simulink model "Scheme"  (R2015a)
settings: Solver=ode45  SolverMode=SingleTasking  StartTime=0.0  StopTime=10  RelTol=1e-3
libraries: simulink x1, dspsrcs4 x1
settings Model: CovSFcnEnable=off  Creator=Olia  LastModifiedBy=Windows 7
settings OptimizationCC: BlockReduction=off  BooleanDataType=off
settings DebuggingCC: SaveWithParameterizedLinksMsg=none  UnderspecifiedInitializationDetection=Classic  MergeDetectMultiDrivingBlocksExec=none  SignalResolutionControl=TryResolveAllWithWarning
settings HardwareCC: TargetUnknown=on

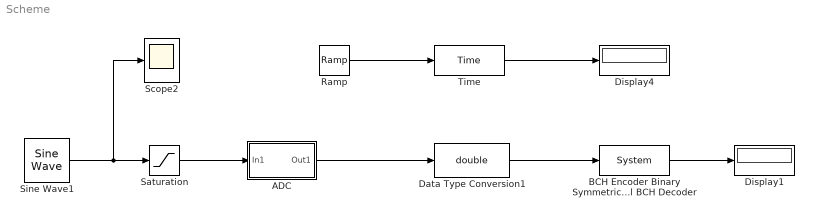
== system Scheme ==
  ADC : Subsystem
  BCH Encoder Binary Symmetric Channel BCH Decoder : MATLABFcn  MATLABFcn=System
  Data Type Conversion1 : DataTypeConversion  OutDataTypeStr=double
  Display1 : Display
  Display4 : Display
  Ramp : simulink/Sources/Ramp  slope=1  start=0  X0=0
  Saturation : Saturate  UpperLimit=2^24-1  LowerLimit=0
  Scope2 : Scope
      settings: TickLabels=on  YMin=0  YMax=10  SaveName=ScopeData2
  Sine Wave1 : dspsrcs4/Sine Wave  Amplitude=10  Frequency=2  Phase=0  SampleMode=Discrete  OutComplex=Real  CompMethod=Trigonometric fcn  TableSize=Speed  SampleTime=1/70  SamplesPerFrame=1  ResetState=Restart at time zero  dataType=double  wordLen=16  udDataType=sfix(16)  fracBitsMode=Best precision  numFracBits=15  OutDataTypeStr=double  LastOutDataTypeStr=double
  Time : MATLABFcn  MATLABFcn=Time
  wires:
  Sine Wave1/1 -> Saturation/1, Scope2/1
  Saturation/1 -> ADC/1(In1)
  ADC/1(Out1) -> Data Type Conversion1/1
  Time/1 -> Display4/1
  Ramp/1 -> Time/1
  Data Type Conversion1/1 -> BCH Encoder Binary Symmetric Channel BCH Decoder/1
  BCH Encoder Binary Symmetric Channel BCH Decoder/1 -> Display1/1

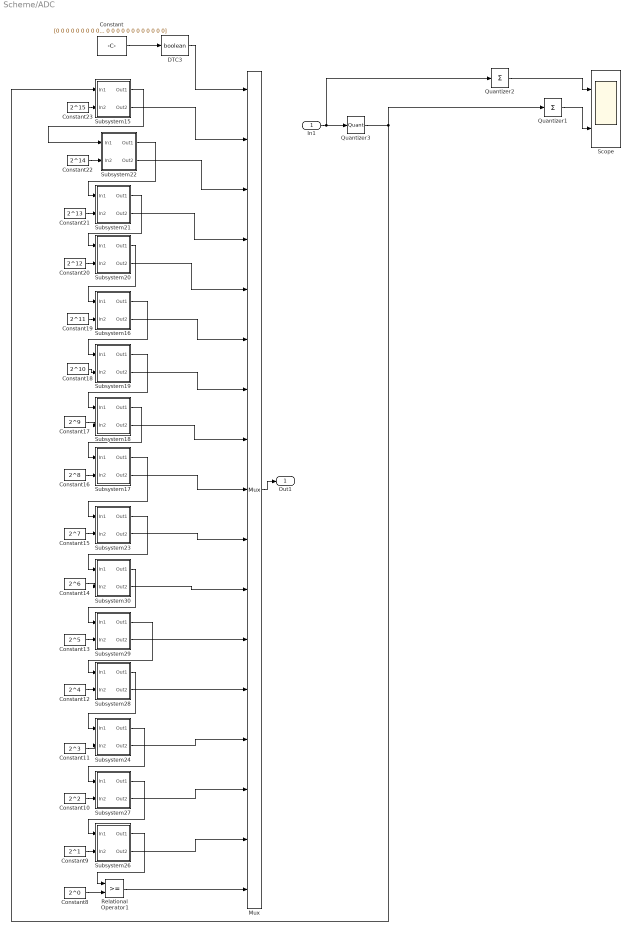
== system Scheme/ADC ==
  In1 : Inport
  Constant : Constant  Value=[0 0 0 0 0 0 0 0 0 0 0 0 0 0 0 0 0 0 0 0 0 0 0 0 0 0 0 0 0 0 0 0 0 0 0 0 0 0 0 0 0 0 0 0 0 0 0 0 0 0 0 0 0 0 0]
  Constant10 : Constant  Value=2^2
  Constant11 : Constant  Value=2^3
  Constant12 : Constant  Value=2^4
  Constant13 : Constant  Value=2^5
  Constant14 : Constant  Value=2^6
  Constant15 : Constant  Value=2^7
  Constant16 : Constant  Value=2^8
  Constant17 : Constant  Value=2^9
  Constant18 : Constant  Value=2^10
  Constant19 : Constant  Value=2^11
  Constant20 : Constant  Value=2^12
  Constant21 : Constant  Value=2^13
  Constant22 : Constant  Value=2^14
  Constant23 : Constant  Value=2^15
  Constant8 : Constant  Value=2^0
  Constant9 : Constant  Value=2^1
  DTC3 : DataTypeConversion  OutDataTypeStr=boolean  LockScale=on
  Mux : Mux  Inputs=17
  Quantizer1 : Sum  Inputs=+
  Quantizer2 : Sum  Inputs=+
  Quantizer3 : Quantizer  QuantizationInterval=0.2
  Relational Operator1 : RelationalOperator  OutDataTypeStr=boolean
  Scope : Scope  NumInputPorts=2
      settings: YMin=-5~-5  YMax=5~5
  Subsystem15 : Subsystem
  Subsystem16 : Subsystem
  Subsystem17 : Subsystem
  Subsystem18 : Subsystem
  Subsystem19 : Subsystem
  Subsystem20 : Subsystem
  Subsystem21 : Subsystem
  Subsystem22 : Subsystem
  Subsystem23 : Subsystem
  Subsystem24 : Subsystem
  Subsystem26 : Subsystem
  Subsystem27 : Subsystem
  Subsystem28 : Subsystem
  Subsystem29 : Subsystem
  Subsystem30 : Subsystem
  Out1 : Outport
  wires:
  Subsystem15/1(Out1) -> Subsystem22/1(In1)
  Quantizer3/1 -> Quantizer1/1, Subsystem15/1(In1)
  Quantizer1/1 -> Scope/2
  Quantizer2/1 -> Scope/1
  Mux/1 -> Out1/1
  In1/1 -> Quantizer2/1, Quantizer3/1
  Subsystem28/1(Out1) -> Subsystem24/1(In1)
  Constant11/1 -> Subsystem24/2(In2)
  Subsystem20/1(Out1) -> Subsystem16/1(In1)
  Subsystem17/1(Out1) -> Subsystem23/1(In1)
  Subsystem26/1(Out1) -> Relational Operator1/1
  Subsystem29/1(Out1) -> Subsystem28/1(In1)
  Subsystem18/1(Out1) -> Subsystem17/1(In1)
  Subsystem21/1(Out1) -> Subsystem20/1(In1)
  Constant22/1 -> Subsystem22/2(In2)
  Constant21/1 -> Subsystem21/2(In2)
  Constant19/1 -> Subsystem16/2(In2)
  Constant20/1 -> Subsystem20/2(In2)
  Constant9/1 -> Subsystem26/2(In2)
  Constant10/1 -> Subsystem27/2(In2)
  Constant12/1 -> Subsystem28/2(In2)
  Constant13/1 -> Subsystem29/2(In2)
  Constant14/1 -> Subsystem30/2(In2)
  Constant15/1 -> Subsystem23/2(In2)
  Constant16/1 -> Subsystem17/2(In2)
  Constant17/1 -> Subsystem18/2(In2)
  Constant18/1 -> Subsystem19/2(In2)
  Constant23/1 -> Subsystem15/2(In2)
  Constant8/1 -> Relational Operator1/2
  Subsystem27/1(Out1) -> Subsystem26/1(In1)
  Subsystem24/1(Out1) -> Subsystem27/1(In1)
  Subsystem30/1(Out1) -> Subsystem29/1(In1)
  Subsystem23/1(Out1) -> Subsystem30/1(In1)
  Subsystem19/1(Out1) -> Subsystem18/1(In1)
  Subsystem16/1(Out1) -> Subsystem19/1(In1)
  Subsystem22/1(Out1) -> Subsystem21/1(In1)
  Relational Operator1/1 -> Mux/17
  Subsystem26/2(Out2) -> Mux/16
  Subsystem27/2(Out2) -> Mux/15
  Subsystem24/2(Out2) -> Mux/14
  Subsystem28/2(Out2) -> Mux/13
  Subsystem29/2(Out2) -> Mux/12
  Subsystem30/2(Out2) -> Mux/11
  Subsystem23/2(Out2) -> Mux/10
  Subsystem17/2(Out2) -> Mux/9
  Subsystem18/2(Out2) -> Mux/8
  Subsystem19/2(Out2) -> Mux/7
  Subsystem16/2(Out2) -> Mux/6
  Subsystem20/2(Out2) -> Mux/5
  Subsystem21/2(Out2) -> Mux/4
  Subsystem22/2(Out2) -> Mux/3
  Subsystem15/2(Out2) -> Mux/2
  Constant/1 -> DTC3/1
  DTC3/1 -> Mux/1

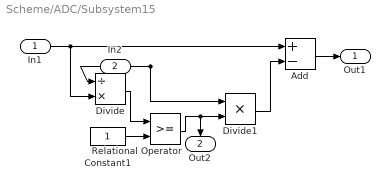
== system Scheme/ADC/Subsystem15 ==
  In1 : Inport
  In2 : Inport  Port=2
  Add : Sum  Inputs=+-
  Constant1 : Constant
  Divide : Product  Inputs=/*
  Divide1 : Product  Inputs=**
  Relational Operator : RelationalOperator  OutDataTypeStr=boolean
  Out1 : Outport
  Out2 : Outport  Port=2
  wires:
  Divide/1 -> Relational Operator/1
  Constant1/1 -> Relational Operator/2
  Relational Operator/1 -> Divide1/2, Out2/1
  Divide1/1 -> Add/2
  In2/1 -> Divide/1, Divide1/1
  In1/1 -> Divide/2, Add/1
  Add/1 -> Out1/1

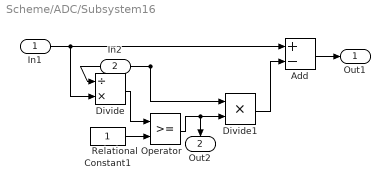
== system Scheme/ADC/Subsystem16 ==
  In1 : Inport
  In2 : Inport  Port=2
  Add : Sum  Inputs=+-
  Constant1 : Constant
  Divide : Product  Inputs=/*
  Divide1 : Product  Inputs=**
  Relational Operator : RelationalOperator  OutDataTypeStr=boolean
  Out1 : Outport
  Out2 : Outport  Port=2
  wires:
  Add/1 -> Out1/1
  In1/1 -> Add/1, Divide/2
  In2/1 -> Divide1/1, Divide/1
  Divide1/1 -> Add/2
  Relational Operator/1 -> Out2/1, Divide1/2
  Constant1/1 -> Relational Operator/2
  Divide/1 -> Relational Operator/1

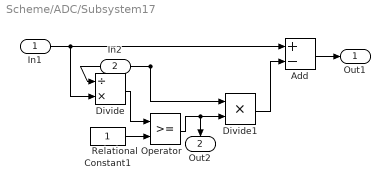
== system Scheme/ADC/Subsystem17 ==
  In1 : Inport
  In2 : Inport  Port=2
  Add : Sum  Inputs=+-
  Constant1 : Constant
  Divide : Product  Inputs=/*
  Divide1 : Product  Inputs=**
  Relational Operator : RelationalOperator  OutDataTypeStr=boolean
  Out1 : Outport
  Out2 : Outport  Port=2
  wires:
  Divide/1 -> Relational Operator/1
  Constant1/1 -> Relational Operator/2
  Relational Operator/1 -> Divide1/2, Out2/1
  Divide1/1 -> Add/2
  In2/1 -> Divide/1, Divide1/1
  In1/1 -> Divide/2, Add/1
  Add/1 -> Out1/1

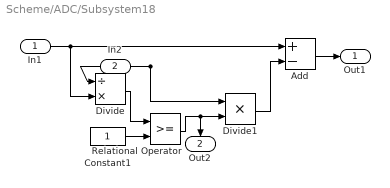
== system Scheme/ADC/Subsystem18 ==
  In1 : Inport
  In2 : Inport  Port=2
  Add : Sum  Inputs=+-
  Constant1 : Constant
  Divide : Product  Inputs=/*
  Divide1 : Product  Inputs=**
  Relational Operator : RelationalOperator  OutDataTypeStr=boolean
  Out1 : Outport
  Out2 : Outport  Port=2
  wires:
  Add/1 -> Out1/1
  In1/1 -> Add/1, Divide/2
  In2/1 -> Divide1/1, Divide/1
  Divide1/1 -> Add/2
  Relational Operator/1 -> Out2/1, Divide1/2
  Constant1/1 -> Relational Operator/2
  Divide/1 -> Relational Operator/1

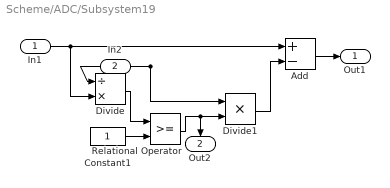
== system Scheme/ADC/Subsystem19 ==
  In1 : Inport
  In2 : Inport  Port=2
  Add : Sum  Inputs=+-
  Constant1 : Constant
  Divide : Product  Inputs=/*
  Divide1 : Product  Inputs=**
  Relational Operator : RelationalOperator  OutDataTypeStr=boolean
  Out1 : Outport
  Out2 : Outport  Port=2
  wires:
  Divide/1 -> Relational Operator/1
  Constant1/1 -> Relational Operator/2
  Relational Operator/1 -> Divide1/2, Out2/1
  Divide1/1 -> Add/2
  In2/1 -> Divide/1, Divide1/1
  In1/1 -> Divide/2, Add/1
  Add/1 -> Out1/1

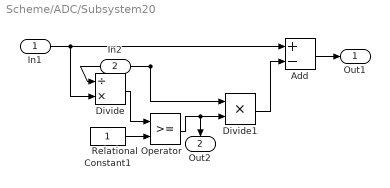
== system Scheme/ADC/Subsystem20 ==
  In1 : Inport
  In2 : Inport  Port=2
  Add : Sum  Inputs=+-
  Constant1 : Constant
  Divide : Product  Inputs=/*
  Divide1 : Product  Inputs=**
  Relational Operator : RelationalOperator  OutDataTypeStr=boolean
  Out1 : Outport
  Out2 : Outport  Port=2
  wires:
  Add/1 -> Out1/1
  In1/1 -> Add/1, Divide/2
  In2/1 -> Divide1/1, Divide/1
  Divide1/1 -> Add/2
  Relational Operator/1 -> Out2/1, Divide1/2
  Constant1/1 -> Relational Operator/2
  Divide/1 -> Relational Operator/1

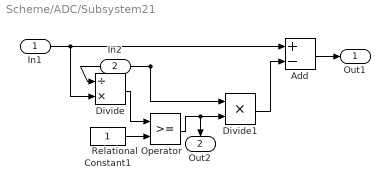
== system Scheme/ADC/Subsystem21 ==
  In1 : Inport
  In2 : Inport  Port=2
  Add : Sum  Inputs=+-
  Constant1 : Constant
  Divide : Product  Inputs=/*
  Divide1 : Product  Inputs=**
  Relational Operator : RelationalOperator  OutDataTypeStr=boolean
  Out1 : Outport
  Out2 : Outport  Port=2
  wires:
  Divide/1 -> Relational Operator/1
  Constant1/1 -> Relational Operator/2
  Relational Operator/1 -> Divide1/2, Out2/1
  Divide1/1 -> Add/2
  In2/1 -> Divide/1, Divide1/1
  In1/1 -> Divide/2, Add/1
  Add/1 -> Out1/1

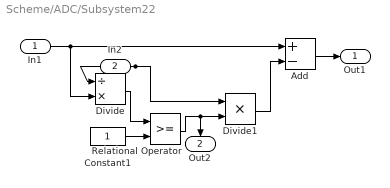
== system Scheme/ADC/Subsystem22 ==
  In1 : Inport
  In2 : Inport  Port=2
  Add : Sum  Inputs=+-
  Constant1 : Constant
  Divide : Product  Inputs=/*
  Divide1 : Product  Inputs=**
  Relational Operator : RelationalOperator  OutDataTypeStr=boolean
  Out1 : Outport
  Out2 : Outport  Port=2
  wires:
  Add/1 -> Out1/1
  In1/1 -> Add/1, Divide/2
  In2/1 -> Divide1/1, Divide/1
  Divide1/1 -> Add/2
  Relational Operator/1 -> Out2/1, Divide1/2
  Constant1/1 -> Relational Operator/2
  Divide/1 -> Relational Operator/1

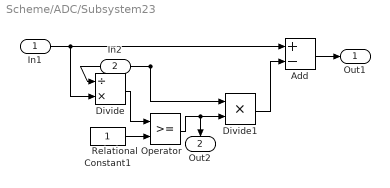
== system Scheme/ADC/Subsystem23 ==
  In1 : Inport
  In2 : Inport  Port=2
  Add : Sum  Inputs=+-
  Constant1 : Constant
  Divide : Product  Inputs=/*
  Divide1 : Product  Inputs=**
  Relational Operator : RelationalOperator  OutDataTypeStr=boolean
  Out1 : Outport
  Out2 : Outport  Port=2
  wires:
  Add/1 -> Out1/1
  In1/1 -> Add/1, Divide/2
  In2/1 -> Divide1/1, Divide/1
  Divide1/1 -> Add/2
  Relational Operator/1 -> Out2/1, Divide1/2
  Constant1/1 -> Relational Operator/2
  Divide/1 -> Relational Operator/1

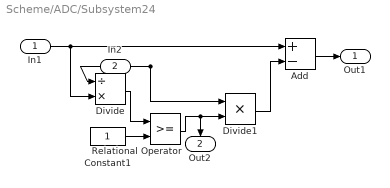
== system Scheme/ADC/Subsystem24 ==
  In1 : Inport
  In2 : Inport  Port=2
  Add : Sum  Inputs=+-
  Constant1 : Constant
  Divide : Product  Inputs=/*
  Divide1 : Product  Inputs=**
  Relational Operator : RelationalOperator  OutDataTypeStr=boolean
  Out1 : Outport
  Out2 : Outport  Port=2
  wires:
  Divide/1 -> Relational Operator/1
  Constant1/1 -> Relational Operator/2
  Relational Operator/1 -> Divide1/2, Out2/1
  Divide1/1 -> Add/2
  In2/1 -> Divide/1, Divide1/1
  In1/1 -> Divide/2, Add/1
  Add/1 -> Out1/1

== system Scheme/ADC/Subsystem26 ==
  In1 : Inport
  In2 : Inport  Port=2
  Add : Sum  Inputs=+-
  Constant1 : Constant
  Divide : Product  Inputs=/*
  Divide1 : Product  Inputs=**
  Relational Operator : RelationalOperator  OutDataTypeStr=boolean
  Out1 : Outport
  Out2 : Outport  Port=2
  wires:
  Divide/1 -> Relational Operator/1
  Constant1/1 -> Relational Operator/2
  Relational Operator/1 -> Divide1/2, Out2/1
  Divide1/1 -> Add/2
  In2/1 -> Divide/1, Divide1/1
  In1/1 -> Divide/2, Add/1
  Add/1 -> Out1/1

== system Scheme/ADC/Subsystem27 ==
  In1 : Inport
  In2 : Inport  Port=2
  Add : Sum  Inputs=+-
  Constant1 : Constant
  Divide : Product  Inputs=/*
  Divide1 : Product  Inputs=**
  Relational Operator : RelationalOperator  OutDataTypeStr=boolean
  Out1 : Outport
  Out2 : Outport  Port=2
  wires:
  Add/1 -> Out1/1
  In1/1 -> Add/1, Divide/2
  In2/1 -> Divide1/1, Divide/1
  Divide1/1 -> Add/2
  Relational Operator/1 -> Out2/1, Divide1/2
  Constant1/1 -> Relational Operator/2
  Divide/1 -> Relational Operator/1

== system Scheme/ADC/Subsystem28 ==
  In1 : Inport
  In2 : Inport  Port=2
  Add : Sum  Inputs=+-
  Constant1 : Constant
  Divide : Product  Inputs=/*
  Divide1 : Product  Inputs=**
  Relational Operator : RelationalOperator  OutDataTypeStr=boolean
  Out1 : Outport
  Out2 : Outport  Port=2
  wires:
  Divide/1 -> Relational Operator/1
  Constant1/1 -> Relational Operator/2
  Relational Operator/1 -> Divide1/2, Out2/1
  Divide1/1 -> Add/2
  In2/1 -> Divide/1, Divide1/1
  In1/1 -> Divide/2, Add/1
  Add/1 -> Out1/1

== system Scheme/ADC/Subsystem29 ==
  In1 : Inport
  In2 : Inport  Port=2
  Add : Sum  Inputs=+-
  Constant1 : Constant
  Divide : Product  Inputs=/*
  Divide1 : Product  Inputs=**
  Relational Operator : RelationalOperator  OutDataTypeStr=boolean
  Out1 : Outport
  Out2 : Outport  Port=2
  wires:
  Add/1 -> Out1/1
  In1/1 -> Add/1, Divide/2
  In2/1 -> Divide1/1, Divide/1
  Divide1/1 -> Add/2
  Relational Operator/1 -> Out2/1, Divide1/2
  Constant1/1 -> Relational Operator/2
  Divide/1 -> Relational Operator/1

== system Scheme/ADC/Subsystem30 ==
  In1 : Inport
  In2 : Inport  Port=2
  Add : Sum  Inputs=+-
  Constant1 : Constant
  Divide : Product  Inputs=/*
  Divide1 : Product  Inputs=**
  Relational Operator : RelationalOperator  OutDataTypeStr=boolean
  Out1 : Outport
  Out2 : Outport  Port=2
  wires:
  Divide/1 -> Relational Operator/1
  Constant1/1 -> Relational Operator/2
  Relational Operator/1 -> Divide1/2, Out2/1
  Divide1/1 -> Add/2
  In2/1 -> Divide/1, Divide1/1
  In1/1 -> Divide/2, Add/1
  Add/1 -> Out1/1
